simulink model "trial"  (R2019b)
settings: Solver=VariableStepAuto  StartTime=0.0  StopTime=5  RelTol=1e-3
model workspace (MAT data in the model file):
  test_model = 1
libraries: dspmathops x3, commchan3 x3
settings Model: Creator=hafizaj  LastModifiedBy=hafizaj

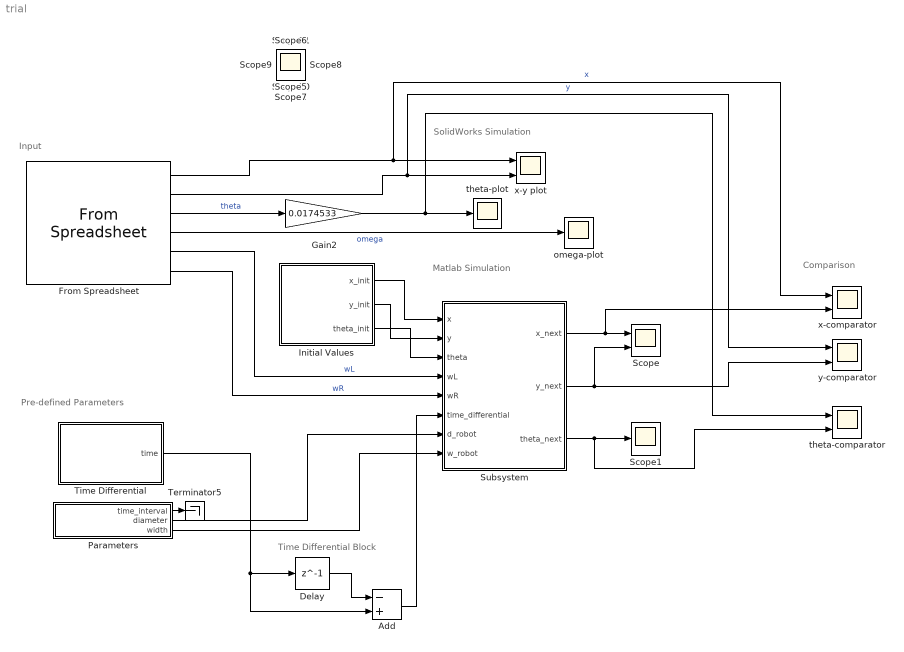
== system trial ==
  note: Comparison
  note: Time Differential Block
  note: SolidWorks Simulation
  note: Input
  note: Pre-defined Parameters
  note: Matlab Simulation
  Add : Sum  Inputs=-+
  Delay : Delay  DelayLength=1  InitialCondition=0
  From Spreadsheet : FromSpreadsheet  FileName=/Users/hafizaj/Desktop/leetCodePractice/ECE183DA/slx_file/Lab 2 Data/Lab2_Segway_Justin.xlsx  SheetName=Sheet2  SampleTime=-1  ExtrapolationBeforeFirstDataPoint=Hold first value  InterpolationWithinTimeRange=Zero order hold  ExtrapolationAfterLastDataPoint=Hold last value
  Gain2 : Gain  Gain=0.0174533
  Initial Values : Subsystem
  Parameters : Subsystem
  Scope : Scope  NumInputPorts=2
  Scope{1..11} (11 alike) : Scope
  Subsystem : Subsystem
  Terminator5 : Terminator
  Time Differential : Subsystem
  omega-plot : Scope
  theta-comparator : Scope  NumInputPorts=2
  theta-plot : Scope
  x-comparator : Scope  NumInputPorts=2
  x-y plot : Scope  NumInputPorts=2
  y-comparator : Scope  NumInputPorts=2
  wires:
  From Spreadsheet/1 -> x-comparator/1, x-y plot/1  "x"
  From Spreadsheet/2 -> x-y plot/2, y-comparator/1  "y"
  From Spreadsheet/3 -> Gain2/1  "theta"
  From Spreadsheet/5 -> Subsystem/4(wL)  "wL"
  From Spreadsheet/6 -> Subsystem/5(wR)  "wR"
  Parameters/2(diameter) -> Subsystem/7(d_robot)
  Parameters/3(width) -> Subsystem/8(w_robot)
  Subsystem/1(x_next) -> x-comparator/2, Scope/1
  Subsystem/2(y_next) -> y-comparator/2, Scope/2
  From Spreadsheet/4 -> omega-plot/1  "omega"
  Delay/1 -> Add/1
  Time Differential/1(time) -> Add/2, Delay/1
  Parameters/1(time_interval) -> Terminator5/1
  Initial Values/1(x_init) -> Subsystem/1(x)
  Initial Values/2(y_init) -> Subsystem/2(y)
  Initial Values/3(theta_init) -> Subsystem/3(theta)
  Subsystem/3(theta_next) -> theta-comparator/2, Scope1/1
  Gain2/1 -> theta-comparator/1, theta-plot/1
  Add/1 -> Subsystem/6(time_differential)

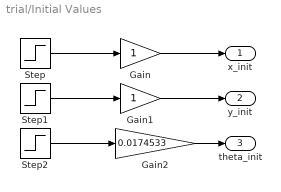
== system trial/Initial Values ==
  Gain : Gain
  Gain1 : Gain
  Gain2 : Gain  Gain=0.0174533
  Step : Step  Time=0  After=8  SampleTime=0
  Step1 : Step  Time=0  After=6  SampleTime=0
  Step2 : Step  Time=0  After=180  SampleTime=0
  x_init : Outport
  y_init : Outport  Port=2
  theta_init : Outport  Port=3
  wires:
  Step2/1 -> Gain2/1
  Step/1 -> Gain/1
  Step1/1 -> Gain1/1
  Gain/1 -> x_init/1
  Gain1/1 -> y_init/1
  Gain2/1 -> theta_init/1

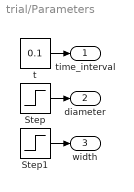
== system trial/Parameters ==
  Step : Step  Time=0  After=0.05  SampleTime=0
  Step1 : Step  Time=0  After=0.09  SampleTime=0
  t : Constant  Value=0.1
  time_interval : Outport
  diameter : Outport  Port=2
  width : Outport  Port=3
  wires:
  t/1 -> time_interval/1
  Step/1 -> diameter/1
  Step1/1 -> width/1

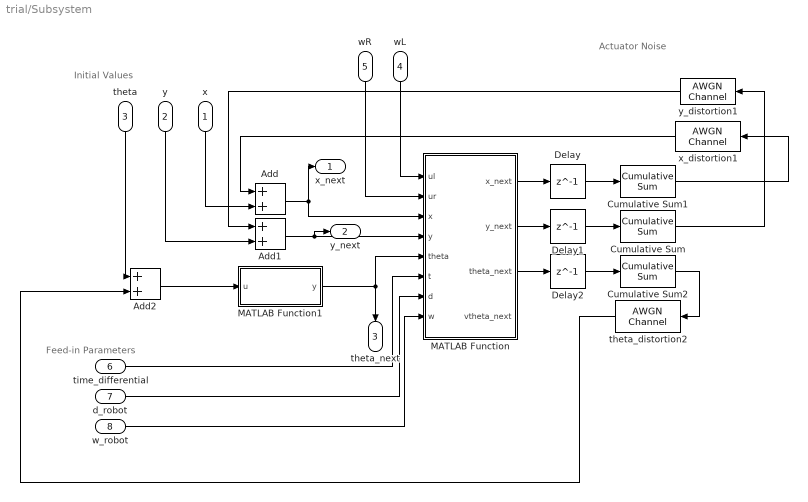
== system trial/Subsystem ==
  note: Initial Values
  note: Feed-in Parameters
  note: Actuator Noise
  x : Inport
  y : Inport  Port=2
  theta : Inport  Port=3
  wL : Inport  Port=4
  wR : Inport  Port=5
  time_differential : Inport  Port=6
  d_robot : Inport  Port=7
  w_robot : Inport  Port=8
  Add : Sum
  Add1 : Sum
  Add2 : Sum
  Cumulative Sum : dspmathops/Cumulative Sum  dim=Channels (running sum)  InputProcessing=Columns as channels (frame based)  reset_popup=None  roundingMode=Floor  overflowMode=off  outputDataTypeStr=Inherit: Same as accumulator  outputMin=[]  outputMax=[]  outputLastDataTypeStr=Inherit: Same as accumulator
      settings: SourceProductName=DSP System Toolbox
  Cumulative Sum1 : dspmathops/Cumulative Sum  dim=Channels (running sum)  InputProcessing=Columns as channels (frame based)  reset_popup=None  roundingMode=Floor  overflowMode=off  outputDataTypeStr=Inherit: Same as accumulator  outputMin=[]  outputMax=[]  outputLastDataTypeStr=Inherit: Same as accumulator
      settings: SourceProductName=DSP System Toolbox
  Cumulative Sum2 : dspmathops/Cumulative Sum  dim=Channels (running sum)  InputProcessing=Columns as channels (frame based)  reset_popup=None  roundingMode=Floor  overflowMode=off  outputDataTypeStr=Inherit: Same as accumulator  outputMin=[]  outputMax=[]  outputLastDataTypeStr=Inherit: Same as accumulator
      settings: SourceProductName=DSP System Toolbox
  Delay : Delay  DelayLength=1  InitialCondition=0
  Delay1 : Delay  DelayLength=1  InitialCondition=0
  Delay2 : Delay  DelayLength=1  InitialCondition=0
  MATLAB Function : MATLAB Function  TreatAsAtomicUnit=on
  MATLAB Function1 : MATLAB Function  TreatAsAtomicUnit=on
  theta_distortion2 : commchan3/AWGN Channel  InputProcessing=Columns as channels (frame based)  seed=67  noiseMode="Signal to noise ratio  (SNR)"  EbNodB=10  EsNodB=10  SNRdB=10  bitsPerSym=1  Ps=0.001  Tsym=1  variance=1
      settings: SourceProductName=Communications Toolbox
  x_distortion1 : commchan3/AWGN Channel  InputProcessing=Columns as channels (frame based)  seed=67  noiseMode="Signal to noise ratio  (SNR)"  EbNodB=10  EsNodB=10  SNRdB=10  bitsPerSym=1  Ps=0.0010  Tsym=1  variance=1
      settings: SourceProductName=Communications Toolbox
  y_distortion1 : commchan3/AWGN Channel  InputProcessing=Columns as channels (frame based)  seed=67  noiseMode="Signal to noise ratio  (SNR)"  EbNodB=10  EsNodB=10  SNRdB=10  bitsPerSym=1  Ps=0.001  Tsym=1  variance=1
      settings: SourceProductName=Communications Toolbox
  x_next : Outport
  y_next : Outport  Port=2
  theta_next : Outport  Port=3
  wires:
  wR/1 -> MATLAB Function/2(ur)
  y/1 -> Add1/2
  wL/1 -> MATLAB Function/1(ul)
  theta/1 -> Add2/1
  MATLAB Function/2(y_next) -> Delay1/1
  time_differential/1 -> MATLAB Function/6(t)
  MATLAB Function/1(x_next) -> Delay/1
  w_robot/1 -> MATLAB Function/8(w)
  x/1 -> Add/2
  d_robot/1 -> MATLAB Function/7(d)
  MATLAB Function/3(theta_next) -> Delay2/1
  Add/1 -> x_next/1, MATLAB Function/3(x)
  Add1/1 -> MATLAB Function/4(y), y_next/1
  Add2/1 -> MATLAB Function1/1(u)
  Delay/1 -> Cumulative Sum1/1
  Delay1/1 -> Cumulative Sum/1
  Delay2/1 -> Cumulative Sum2/1
  MATLAB Function1/1(y) -> MATLAB Function/5(theta), theta_next/1
  Cumulative Sum/1 -> y_distortion1/1
  Cumulative Sum1/1 -> x_distortion1/1
  Cumulative Sum2/1 -> theta_distortion2/1
  y_distortion1/1 -> Add1/1
  x_distortion1/1 -> Add/1
  theta_distortion2/1 -> Add2/2

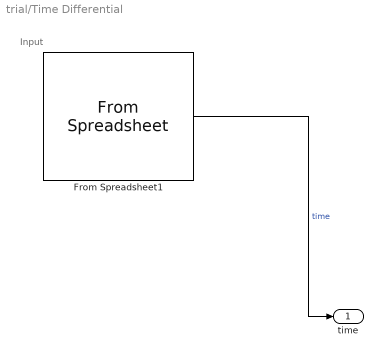
== system trial/Time Differential ==
  note: Input
  From Spreadsheet1 : FromSpreadsheet  FileName=/Users/hafizaj/Desktop/leetCodePractice/ECE183DA/slx_file/Lab 2 Data/Lab2_Segway_Justin.xlsx  SheetName=Sheet3  SampleTime=-1  ExtrapolationBeforeFirstDataPoint=Hold first value  InterpolationWithinTimeRange=Zero order hold  ExtrapolationAfterLastDataPoint=Hold last value
  time : Outport
  wires:
  From Spreadsheet1/1 -> time/1  "time"

== matlab function trial/Subsystem/MATLAB Function1 ==
  data: u input; y output
function y = fcn(u)

y = (u - 2*pi*floor( (u+pi)/(2*pi) ))

== matlab function trial/Subsystem/MATLAB Function ==
  data: ul input; x_next output; ur input; x input; y input; theta input; t input; d input; w input; y_next output; theta_next output; vtheta_next output
function [x_next, y_next, theta_next, vtheta_next] = fcn(ul, ur, x, y, theta, t,d,w)
    
    %Define the state space equation
    ydot = 0.25*d*cos(theta)*ul + 0.25*d*cos(theta)*ur;
    xdot = 0.25*d*sin(theta)*ul + 0.25*d*sin(theta)*ur;
    thetadot = (d/(2*w))*ul - (d/(2*w))*ur;
    
    
    %Calculate the next state
    x_next = xdot*t;
    y_next = ydot*t;
    theta_next = thetadot*t;
    vtheta_next = thetadot;
end
